simulink model "analisis"  (R2018a)
settings: Solver=ode45  StartTime=0.0  StopTime=70  MaxStep=1e-4  RelTol=1e-3
undefined symbols (not defined in the file): wn
settings Model: Creator=carma  LastModifiedBy=carma

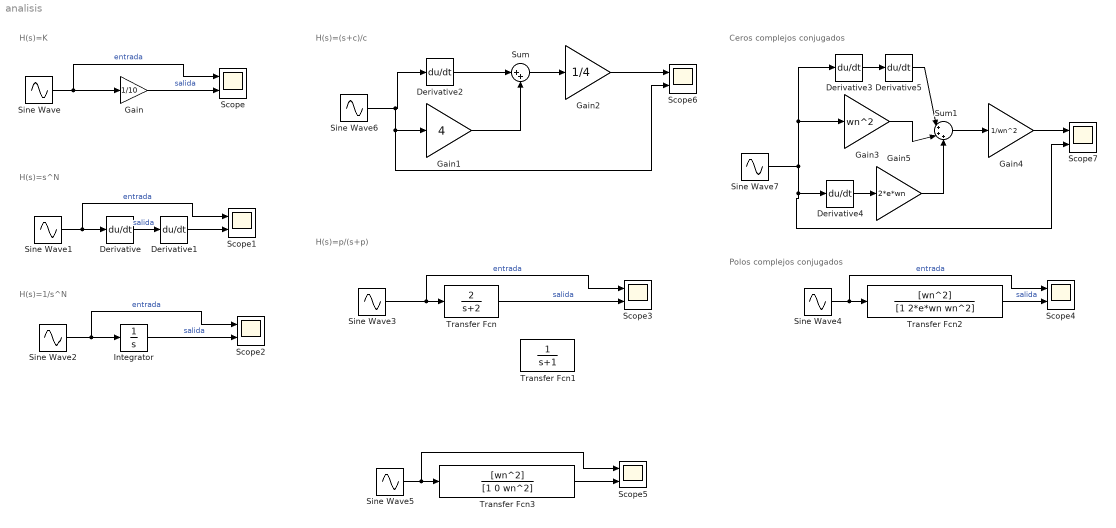
== system analisis ==
  note: Polos complejos conjugados
  note: Ceros complejos conjugados
  note: H(s)=p/(s+p)
  note: H(s)=(s+c)/c
  note: H(s)=1/s^N
  note: H(s)=s^N
  note: H(s)=K
  Derivative{,1..5} (6 alike) : Derivative  CoefficientInTFapproximation=0
  Gain : Gain  Gain=1/10
  Gain1 : Gain  Gain=4
  Gain2 : Gain  Gain=1/4
  Gain3 : Gain  Gain=wn^2
  Gain4 : Gain  Gain=1/wn^2
  Gain5 : Gain  Gain=2*e*wn
  Integrator : Integrator
  Scope{,1..7} (8 alike) : Scope  NumInputPorts=2
  Sine Wave : Sin  Frequency=100  Phase=pi/4  SampleTime=0
  Sine Wave1 : Sin  SampleTime=0
  Sine Wave2 : Sin  Frequency=0.1  SampleTime=0
  Sine Wave3 : Sin  Frequency=0.01  SampleTime=0
  Sine Wave4 : Sin  Frequency=wn*sqrt(1-2*e^2)  SampleTime=0
  Sine Wave5 : Sin  Frequency=wn  SampleTime=0
  Sine Wave6 : Sin  Frequency=100  SampleTime=0
  Sine Wave7 : Sin  Frequency=0.01  SampleTime=0
  Sum : Sum  Inputs=|++
  Sum1 : Sum  Inputs=|+++
  Transfer Fcn : TransferFcn  Numerator=[2]  Denominator=[1 2]
  Transfer Fcn1 : TransferFcn  Denominator=[1 1]
  Transfer Fcn2 : TransferFcn  Numerator=[wn^2]  Denominator=[1 2*e*wn wn^2]
  Transfer Fcn3 : TransferFcn  Numerator=[wn^2]  Denominator=[1 0 wn^2]
  wires:
  Sine Wave/1 -> Scope/1, Gain/1  "entrada"
  Gain/1 -> Scope/2  "salida"
  Derivative/1 -> Derivative1/1  "salida"
  Sine Wave1/1 -> Derivative/1, Scope1/1  "entrada"
  Integrator/1 -> Scope2/2  "salida"
  Sine Wave2/1 -> Integrator/1, Scope2/1  "entrada"
  Sine Wave3/1 -> Transfer Fcn/1, Scope3/1  "entrada"
  Transfer Fcn/1 -> Scope3/2  "salida"
  Sine Wave4/1 -> Scope4/1, Transfer Fcn2/1  "entrada"
  Transfer Fcn2/1 -> Scope4/2  "salida"
  Sine Wave5/1 -> Scope5/1, Transfer Fcn3/1
  Transfer Fcn3/1 -> Scope5/2
  Derivative2/1 -> Sum/1
  Gain1/1 -> Sum/2
  Sine Wave6/1 -> Scope6/2, Gain1/1, Derivative2/1
  Sum/1 -> Gain2/1
  Gain2/1 -> Scope6/1
  Gain3/1 -> Sum1/2
  Derivative3/1 -> Derivative5/1
  Sum1/1 -> Gain4/1
  Gain4/1 -> Scope7/1
  Sine Wave7/1 -> Gain3/1, Derivative3/1, Scope7/2, Derivative4/1
  Derivative5/1 -> Sum1/1
  Derivative4/1 -> Gain5/1
  Gain5/1 -> Sum1/3
  Derivative1/1 -> Scope1/2
